simulink library "lib_mtpa_reference_current_generator"  (R2023a)
settings: Solver=VariableStepAuto  StartTime=0.0  StopTime=10.0  RelTol=1e-3
libraries: lib_conversion x14, lib_dynamic_saturator x2, lib_square_root x2, simulink x1
settings Model: Creator=cav2ofo  LastModifiedBy=lenovo
settings OptimizationCC: ReuseModelBlockBuffer=off

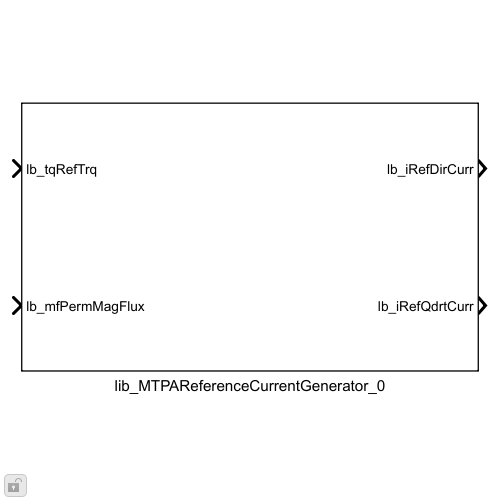
[thumbnail: Simulink's stored preview of the top-level diagram]
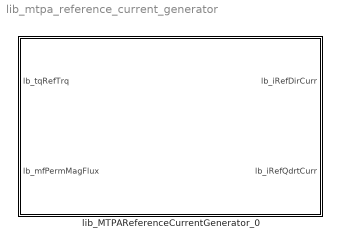
== system lib_mtpa_reference_current_generator ==
  lib_MTPAReferenceCurrentGenerator_0 : Subsystem  mask{lb_parPolePairNum=5, lb_parPermMagFlux=2e-3, lb_parMagTempCoef=-1e-3, lb_parDirIndc=1e-5, lb_parQdrtIndc=1e-5, lb_parMaxPhsCurr=50, lb_parDmgzFact=1, lb_parMaxOperTrq=1, lb_parMinOperTrq=-1, lb_parTrqSampNum=60, lb_parMaxOperTemp=140, lb_parMinOperTemp=-20, lb_parTempSampNum=20, lb_parOutpDataType=Inherit: Inherit via back propagation}
      mask prompts: lb_parPolePairNum "Pole pairs number [-]:"; lb_parPermMagFlux "Permanent magnet flux at 20[oC]:"; lb_parMagTempCoef "Magnet temperature coefficient [1/K]:"; lb_parDirIndc "Direct inductance [H]:"; lb_parQdrtIndc "Quadrature inductance [H]:"; lb_parMaxPhsCurr "Maximum phase current [A]:"; lb_parDmgzFact "Demagnetization factor [-]:"; lb_parMaxOperTrq "Maximum operating torque [Nm]:"; lb_parMinOperTrq "Minimum operating torque [Nm]:"; lb_parTrqSampNum "Torque samplings number:"; lb_parMaxOperTemp "Maximum operating temperature [oC]:"; lb_parMinOperTemp "Minimum operating temperature [oC]:"; lb_parTempSampNum "Temperature samplings number:"; lb_parOutpDataType "Output data type:"
      mask init:
      | temp.PermMagFlux_scl = double(lb_parPermMagFlux);  % [Vs] Permanent magnet flux at 20°C
      | temp.Ld_scl = double(lb_parDirIndc);  % [H] Direct inductance
      | temp.Lq_scl = double(lb_parQdrtIndc);  % [H] Quadrature inductance
      | temp.Npp_scl = double(lb_parPolePairNum);  % Number of pole pairs
      | temp.TmpCoeff_scl = double(lb_parMagTempCoef);  % [1/K] Temperature coefficient of permanent magnet
      | temp.IPhaseMax_scl = double(lb_parMaxPhsCurr);  % [A] Max phase current
      | 
      | % Define torque data
      | temp.Trq_arr = linspace(lb_parMinOperTrq,lb_parMaxOperTrq,lb_parTrqSampNum);  % [Nm] Reference values of electric torque
      | temp.NewTrqStep_scl = 2^(ceil(log2((lb_parMaxOperTrq-lb_parMinOperTrq)/(lb_parTrqSampNum-1))));
      | temp.NewMaxTrq_scl = lb_parMinOperTrq + temp.NewTrqStep_scl*(lb_parTrqSampNum-1);
      | temp.Trq_arr = (lb_parMinOperTrq:temp.NewTrqStep_scl:temp.NewMaxTrq_scl);
      | 
      | % Define temperature/permanent magnet flux data
      | temp.MaxPermMagFlux_scl = temp.PermMagFlux_scl*(1+temp.TmpCoeff_scl*(lb_parMinOperTemp-20));
      | temp.MinPermMagFlux_scl = temp.PermMagFlux_scl*(1+temp.TmpCoeff_scl*(lb_parMaxOperTemp-20));
      | temp.PermMagFlux_arr = linspace(temp.MinPermMagFlux_scl,temp.MaxPermMagFlux_scl,lb_parTempSampNum);
      | temp.NewPermMagFluxStep_scl = 2^(ceil(log2((temp.MaxPermMagFlux_scl-temp.MinPermMagFlux_scl)/(lb_parTempSampNum-1))));
      | temp.NewMaxPermMagFlux_scl = temp.MinPermMagFlux_scl + temp.NewPermMagFluxStep_scl*(lb_parTempSampNum-1);
      | temp.PermMagFlux_arr = linspace(temp.MinPermMagFlux_scl,temp.NewMaxPermMagFlux_scl,lb_parTempSampNum);
      | 
      | temp.IdMTPA_mat = zeros(lb_parTrqSampNum,lb_parTempSampNum);  % [A] Initialization of MTPA LUT
      | 
      | 
      | 
      | for ii = 1:lb_parTrqSampNum
      | 
      |     for jj = 1:lb_parTempSampNum
      | 
      |         % The following quartic equation represents the Maximum Torque Per Ampere
      |         % control strategy. The solution returns the direct current adsdsadsdds
      |         % corresponding to a given electric torque.
      | 
      |         temp.idMTPA_fun = @(id) 1e10*(9*temp.Npp_scl^2*(temp.Lq_scl-temp.Ld_scl)^3*id.^4 + ...
      |             - 27*temp.Npp_scl^2*temp.PermMagFlux_arr(jj)*(temp.Lq_scl-temp.Ld_scl)^2*id.^3 + ...
      |             27*temp.Npp_scl^2*temp.PermMagFlux_arr(jj)^2*(temp.Lq_scl-temp.Ld_scl)*id.^2 + ...
      |             - 9*temp.Npp_scl^2*temp.PermMagFlux_arr(jj)^3*id + ...
      |             - 4*(temp.Lq_scl-temp.Ld_scl)*temp.Trq_arr(ii)^2);
      | 
      |         if jj == 1 || jj == 2
      |             temp.IdMTPA_mat(ii,jj) = real(fzero(temp.idMTPA_fun,-1e-1));
      |         else
      |             temp.IdMTPA_mat(ii,jj) = fzero(temp.idMTPA_fun,temp.IdMTPA_mat(ii,jj-1));
      |         end
      | 
      |     end
      | end
      | 
      | lb_parMTPATrqDataFrstVal = temp.Trq_arr(1);
      | lb_parMTPATrqDataStepVal = temp.NewTrqStep_scl;
      | lb_parMTPAPermMagFluxDataFrstVal = temp.PermMagFlux_arr(1);
      | lb_parMTPAPermMagFluxDataStepVal = temp.NewPermMagFluxStep_scl;
      | lb_parMTPA2DLktMtrx = temp.IdMTPA_mat;
      | 
      | 
      | 
      | clear temp
      settings: LibrarySourceBlock=lib_reference_current_generator/lib_ReferenceCurrentGenerator_0
      mask DialogControl DescGroupVar Prompt: VHIT control library
      mask DialogControl DescTextVar Prompt: Reference current generator
      mask DialogControl Container4 Prompt: Lookup table parameters
      mask DialogControl Container3 Prompt: Data type

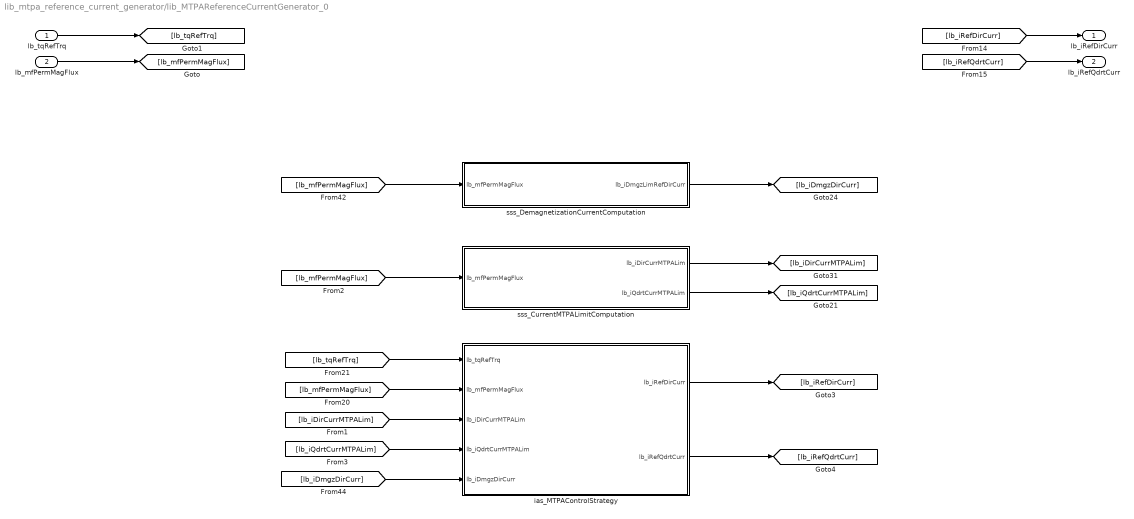
== system lib_mtpa_reference_current_generator/lib_MTPAReferenceCurrentGenerator_0 ==
  lb_tqRefTrq : Inport
  lb_mfPermMagFlux : Inport  Port=2
  ias_MTPAControlStrategy : Subsystem  TreatAsAtomicUnit=on
  sss_CurrentMTPALimitComputation : Subsystem
  sss_DemagnetizationCurrentComputation : Subsystem
  lb_iRefDirCurr : Outport
  lb_iRefQdrtCurr : Outport  Port=2
  wires:
  [lb_mfPermMagFlux] -> sss_DemagnetizationCurrentComputation/1(lb_mfPermMagFlux)
  lb_mfPermMagFlux/1 -> [lb_mfPermMagFlux]
  ias_MTPAControlStrategy/1(lb_iRefDirCurr) -> [lb_iRefDirCurr]
  lb_tqRefTrq/1 -> [lb_tqRefTrq]
  [lb_iRefDirCurr] -> lb_iRefDirCurr/1
  [lb_mfPermMagFlux] -> ias_MTPAControlStrategy/2(lb_mfPermMagFlux)
  [lb_iDirCurrMTPALim] -> ias_MTPAControlStrategy/3(lb_iDirCurrMTPALim)
  ias_MTPAControlStrategy/2(lb_iRefQdrtCurr) -> [lb_iRefQdrtCurr]
  sss_CurrentMTPALimitComputation/2(lb_iQdrtCurrMTPALim) -> [lb_iQdrtCurrMTPALim]
  [lb_iRefQdrtCurr] -> lb_iRefQdrtCurr/1
  [lb_tqRefTrq] -> ias_MTPAControlStrategy/1(lb_tqRefTrq)
  sss_CurrentMTPALimitComputation/1(lb_iDirCurrMTPALim) -> [lb_iDirCurrMTPALim]
  [lb_iQdrtCurrMTPALim] -> ias_MTPAControlStrategy/4(lb_iQdrtCurrMTPALim)
  [lb_mfPermMagFlux] -> sss_CurrentMTPALimitComputation/1(lb_mfPermMagFlux)
  [lb_iDmgzDirCurr] -> ias_MTPAControlStrategy/5(lb_iDmgzDirCurr)
  sss_DemagnetizationCurrentComputation/1(lb_iDmgzLimRefDirCurr) -> [lb_iDmgzDirCurr]

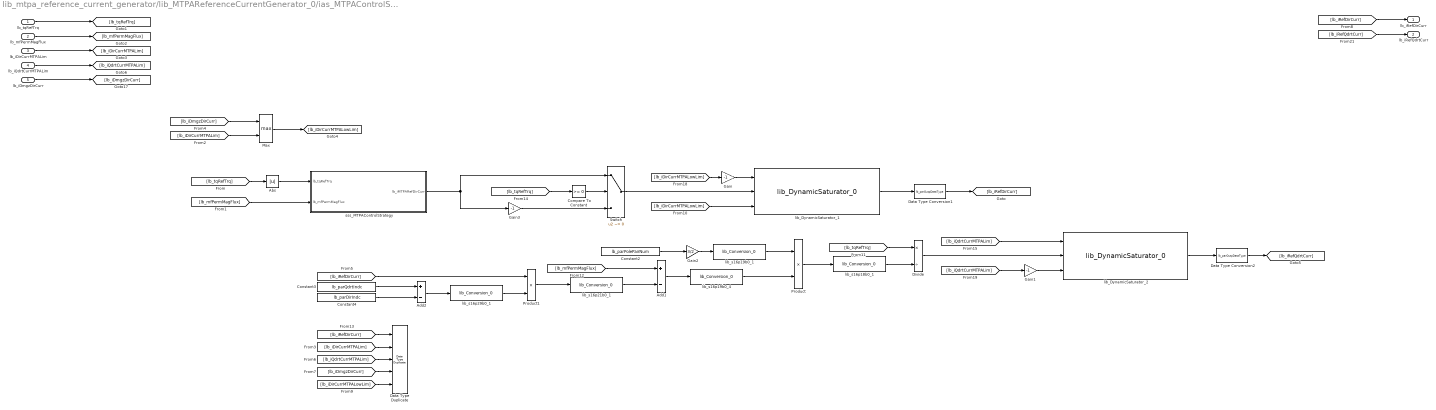
== system lib_mtpa_reference_current_generator/lib_MTPAReferenceCurrentGenerator_0/ias_MTPAControlStrategy ==
  lb_tqRefTrq : Inport
  lb_mfPermMagFlux : Inport  Port=2
  lb_iDirCurrMTPALim : Inport  Port=3
  lb_iQdrtCurrMTPALim : Inport  Port=4
  lb_iDmgzDirCurr : Inport  Port=5
  Abs : Abs  SaturateOnIntegerOverflow=off
  Add1 : Sum  Inputs=+-  OutDataTypeStr=Inherit: Inherit via back propagation  RndMeth=Simplest
  Add2 : Sum  Inputs=+-  OutDataTypeStr=Inherit: Inherit via back propagation  RndMeth=Simplest
  Compare To Constant : simulink/Logic and Bit Operations/Compare To Constant  relop=>=  const=0  OutDataTypeStr=boolean
  Constant2 : Constant  Value=lb_parPolePairNum
  Constant3 : Constant  Value=lb_parQdrtIndc
  Constant4 : Constant  Value=lb_parDirIndc
  Data Type Duplicate : DataTypeDuplicate  NumInputPorts=5
  Data Type Conversion1 : DataTypeConversion  OutDataTypeStr=lb_parOutpDataType  SaturateOnIntegerOverflow=off  RndMeth=Floor
  Data Type Conversion2 : DataTypeConversion  OutDataTypeStr=lb_parOutpDataType  SaturateOnIntegerOverflow=off  RndMeth=Floor
  Divide : Product  Inputs=*/  OutDataTypeStr=Inherit: Inherit via back propagation  RndMeth=Simplest
  Gain : Gain  Gain=-1  OutDataTypeStr=Inherit: Inherit via back propagation  RndMeth=Simplest
  Gain1 : Gain  Gain=-1  OutDataTypeStr=Inherit: Inherit via back propagation  RndMeth=Simplest
  Gain2 : Gain  Gain=3/2  OutDataTypeStr=Inherit: Inherit via back propagation  RndMeth=Simplest
  Gain3 : Gain  Gain=-1  OutDataTypeStr=Inherit: Same as input
  Max : MinMax  Function=max  Inputs=2  OutDataTypeStr=Inherit: Inherit via back propagation
  Product : Product  OutDataTypeStr=Inherit: Inherit via back propagation  RndMeth=Simplest
  Product1 : Product  OutDataTypeStr=Inherit: Inherit via back propagation  RndMeth=Simplest
  Switch : Switch  Criteria=u2 ~= 0  SaturateOnIntegerOverflow=off  InputSameDT=off
  lib_DynamicSaturator_1 : lib_dynamic_saturator/lib_DynamicSaturator_0
  lib_DynamicSaturator_2 : lib_dynamic_saturator/lib_DynamicSaturator_0
  lib_s16p18b0_1 : lib_conversion/lib_Conversion_0  lb_parDataType=fixdt(1,16,2^-18,0)  lb_parOutpMaxVal=[]  lb_parOutpMinVal=[]  lb_parSatFlag=off
  lib_s16p19b0_1 : lib_conversion/lib_Conversion_0  lb_parDataType=fixdt(0,16,10^-3,0)  lb_parOutpMaxVal=[]  lb_parOutpMinVal=[]  lb_parSatFlag=off
  lib_s16p19b0_4 : lib_conversion/lib_Conversion_0  lb_parDataType=fixdt(1,16,2^-19,0)  lb_parOutpMaxVal=[]  lb_parOutpMinVal=[]  lb_parSatFlag=off
  lib_s16p21b0_1 : lib_conversion/lib_Conversion_0  lb_parDataType=fixdt(1,16,2^-21,0)  lb_parOutpMaxVal=[]  lb_parOutpMinVal=[]  lb_parSatFlag=off
  lib_s16p29b0_1 : lib_conversion/lib_Conversion_0  lb_parDataType=fixdt(1,16,2^-29,0)  lb_parOutpMaxVal=[]  lb_parOutpMinVal=[]  lb_parSatFlag=off
  sss_MTPAControlStrategy : Subsystem
  lb_iRefDirCurr : Outport
  lb_iRefQdrtCurr : Outport  Port=2
  wires:
  [lb_iRefDirCurr] -> Data Type Duplicate/1
  [lb_iDirCurrMTPALowLim] -> Data Type Duplicate/5
  [lb_iQdrtCurrMTPALim] -> Data Type Duplicate/3
  [lb_iDmgzDirCurr] -> Data Type Duplicate/4
  [lb_iDirCurrMTPALim] -> Data Type Duplicate/2
  [lb_iRefDirCurr] -> lb_iRefDirCurr/1
  [lb_iRefQdrtCurr] -> lb_iRefQdrtCurr/1
  lib_s16p19b0_1/1 -> Product/1
  Gain2/1 -> lib_s16p19b0_1/1
  lb_tqRefTrq/1 -> [lb_tqRefTrq]
  lb_mfPermMagFlux/1 -> [lb_mfPermMagFlux]
  [lb_tqRefTrq] -> Abs/1
  [lb_mfPermMagFlux] -> sss_MTPAControlStrategy/2(lb_mfPermMagFlux)
  [lb_iDirCurrMTPALowLim] -> Gain/1
  lib_DynamicSaturator_1/1 -> Data Type Conversion1/1
  Data Type Conversion1/1 -> [lb_iRefDirCurr]
  Product/1 -> lib_s16p18b0_1/1
  lib_s16p19b0_4/1 -> Product/2
  Add1/1 -> lib_s16p19b0_4/1
  lib_s16p21b0_1/1 -> Add1/2
  lib_s16p18b0_1/1 -> Divide/2
  lib_s16p29b0_1/1 -> Product1/2
  Product1/1 -> lib_s16p21b0_1/1
  [lb_tqRefTrq] -> Divide/1
  [lb_mfPermMagFlux] -> Add1/1
  [lb_iRefDirCurr] -> Product1/1
  Constant3/1 -> Add2/1
  Constant2/1 -> Gain2/1
  Constant4/1 -> Add2/2
  Add2/1 -> lib_s16p29b0_1/1
  [lb_iQdrtCurrMTPALim] -> Gain1/1
  Data Type Conversion2/1 -> [lb_iRefQdrtCurr]
  lib_DynamicSaturator_2/1 -> Data Type Conversion2/1
  [lb_iQdrtCurrMTPALim] -> lib_DynamicSaturator_2/1
  Divide/1 -> lib_DynamicSaturator_2/2
  lb_iDirCurrMTPALim/1 -> [lb_iDirCurrMTPALim]
  lb_iQdrtCurrMTPALim/1 -> [lb_iQdrtCurrMTPALim]
  lb_iDmgzDirCurr/1 -> [lb_iDmgzDirCurr]
  [lb_iDirCurrMTPALim] -> Max/2
  [lb_iDmgzDirCurr] -> Max/1
  Max/1 -> [lb_iDirCurrMTPALowLim]
  [lb_iDirCurrMTPALowLim] -> lib_DynamicSaturator_1/3
  Gain/1 -> lib_DynamicSaturator_1/1
  Gain1/1 -> lib_DynamicSaturator_2/3
  Abs/1 -> sss_MTPAControlStrategy/1(lb_tqRefTrq)
  [lb_tqRefTrq] -> Compare To Constant/1
  Compare To Constant/1 -> Switch/2
  Gain3/1 -> Switch/3
  Switch/1 -> lib_DynamicSaturator_1/2
  sss_MTPAControlStrategy/1(lb_iMTPARefDirCurr) -> Gain3/1, Switch/1

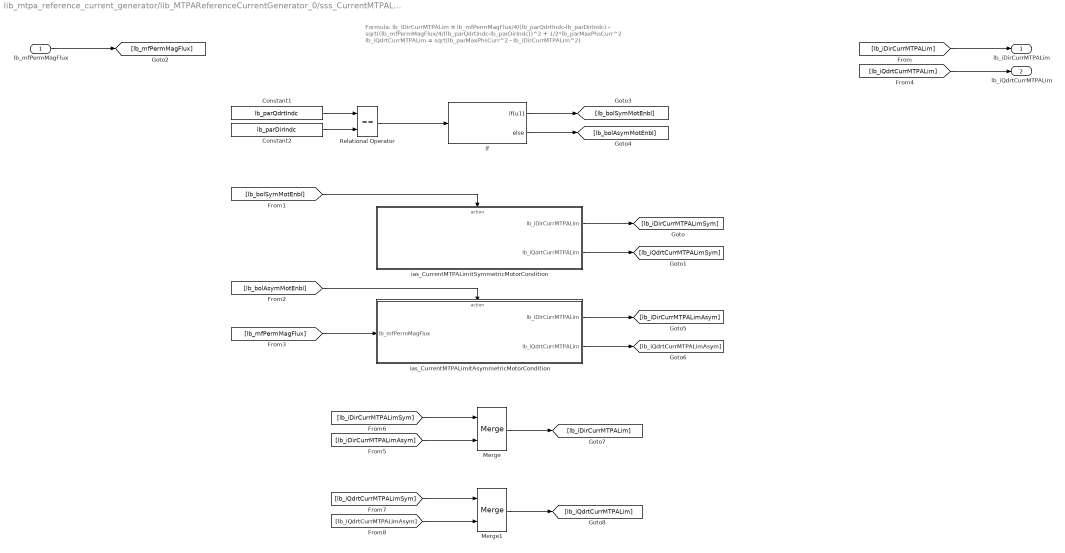
== system lib_mtpa_reference_current_generator/lib_MTPAReferenceCurrentGenerator_0/sss_CurrentMTPALimitComputation ==
  note: Formula:
      | lb_iDirCurrMTPALim = lb_mfPermMagFlux/4/(lb_parQdrtIndc-lb_parDirIndc) - sqrt((lb_mfPermMagFlux/4/(lb_parQdrtIndc-lb_parDirIndc))^2 + 1/2*lb_parMaxPhsCurr^2
      | lb_iQdrtCurrMTPALim = sqrt(lb_parMaxPhsCurr^2 - lb_iDirCurrMTPALim^2)
  lb_mfPermMagFlux : Inport
  Constant1 : Constant  Value=lb_parQdrtIndc
  Constant2 : Constant  Value=lb_parDirIndc
  If : If  IfExpression=u1
  Merge : Merge
  Merge1 : Merge
  Relational Operator : RelationalOperator  Operator===  OutDataTypeStr=boolean  RndMeth=Simplest  InputSameDT=off
  ias_CurrentMTPALimitAsymmetricMotorCondition : Subsystem  TreatAsAtomicUnit=on
  ias_CurrentMTPALimitSymmetricMotorCondition : Subsystem  TreatAsAtomicUnit=on
  lb_iDirCurrMTPALim : Outport
  lb_iQdrtCurrMTPALim : Outport  Port=2
  wires:
  Merge1/1 -> [lb_iQdrtCurrMTPALim]
  Merge/1 -> [lb_iDirCurrMTPALim]
  [lb_iQdrtCurrMTPALimAsym] -> Merge1/2
  [lb_iQdrtCurrMTPALimSym] -> Merge1/1
  [lb_iDirCurrMTPALimSym] -> Merge/1
  [lb_iDirCurrMTPALimAsym] -> Merge/2
  [lb_mfPermMagFlux] -> ias_CurrentMTPALimitAsymmetricMotorCondition/1(lb_mfPermMagFlux)
  ias_CurrentMTPALimitAsymmetricMotorCondition/2(lb_iQdrtCurrMTPALim) -> [lb_iQdrtCurrMTPALimAsym]
  ias_CurrentMTPALimitAsymmetricMotorCondition/1(lb_iDirCurrMTPALim) -> [lb_iDirCurrMTPALimAsym]
  ias_CurrentMTPALimitSymmetricMotorCondition/2(lb_iQdrtCurrMTPALim) -> [lb_iQdrtCurrMTPALimSym]
  ias_CurrentMTPALimitSymmetricMotorCondition/1(lb_iDirCurrMTPALim) -> [lb_iDirCurrMTPALimSym]
  [lb_bolAsymMotEnbl] -> ias_CurrentMTPALimitAsymmetricMotorCondition/Action
  [lb_bolSymMotEnbl] -> ias_CurrentMTPALimitSymmetricMotorCondition/Action
  If/2 -> [lb_bolAsymMotEnbl]
  If/1 -> [lb_bolSymMotEnbl]
  Relational Operator/1 -> If/1
  Constant2/1 -> Relational Operator/2
  Constant1/1 -> Relational Operator/1
  [lb_iDirCurrMTPALim] -> lb_iDirCurrMTPALim/1
  [lb_iQdrtCurrMTPALim] -> lb_iQdrtCurrMTPALim/1
  lb_mfPermMagFlux/1 -> [lb_mfPermMagFlux]

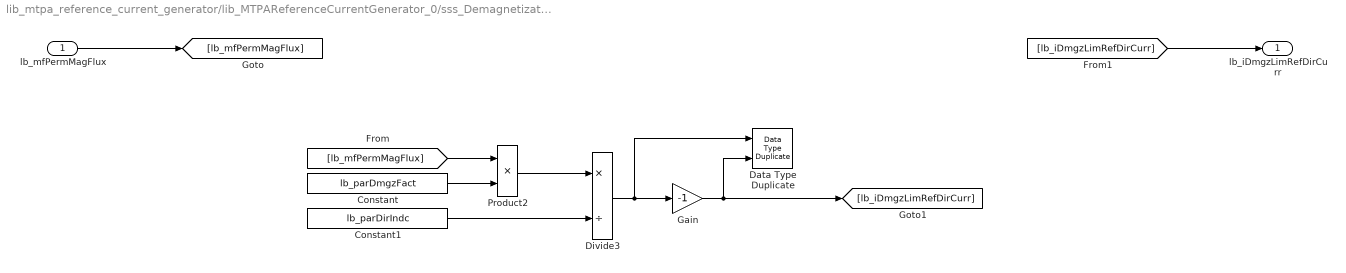
== system lib_mtpa_reference_current_generator/lib_MTPAReferenceCurrentGenerator_0/sss_DemagnetizationCurrentComputation ==
  lb_mfPermMagFlux : Inport
  Constant : Constant  Value=lb_parDmgzFact
  Constant1 : Constant  Value=lb_parDirIndc
  Data Type Duplicate : DataTypeDuplicate
  Divide3 : Product  Inputs=*/  OutDataTypeStr=Inherit: Inherit via back propagation  RndMeth=Simplest
  Gain : Gain  Gain=-1  OutDataTypeStr=Inherit: Inherit via back propagation  RndMeth=Simplest
  Product2 : Product  RndMeth=Simplest  OutDataTypeStr=Inherit: Same as first input
  lb_iDmgzLimRefDirCurr : Outport
  wires:
  Divide3/1 -> Gain/1, Data Type Duplicate/1
  Product2/1 -> Divide3/1
  [lb_mfPermMagFlux] -> Product2/1
  Gain/1 -> [lb_iDmgzLimRefDirCurr], Data Type Duplicate/2
  Constant/1 -> Product2/2
  lb_mfPermMagFlux/1 -> [lb_mfPermMagFlux]
  [lb_iDmgzLimRefDirCurr] -> lb_iDmgzLimRefDirCurr/1
  Constant1/1 -> Divide3/2

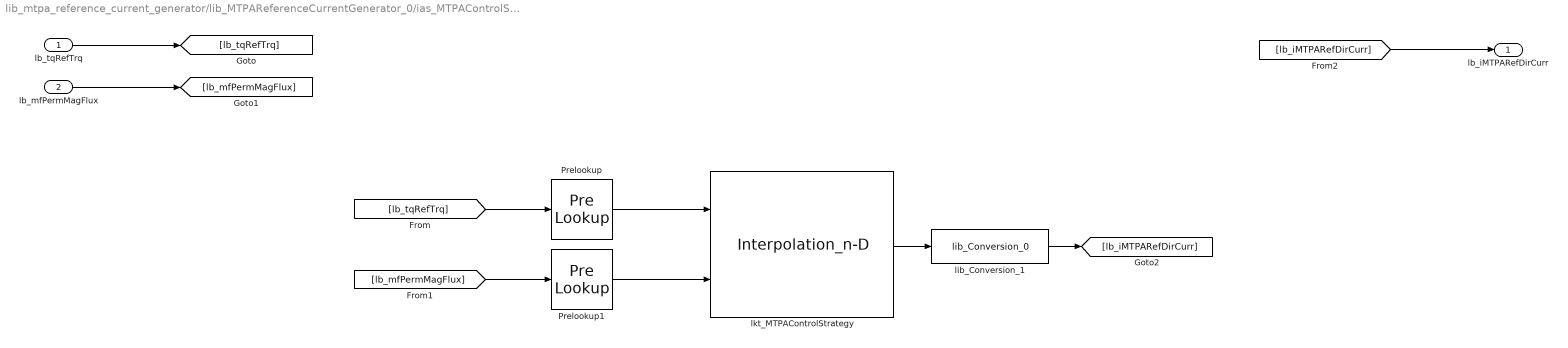
== system lib_mtpa_reference_current_generator/lib_MTPAReferenceCurrentGenerator_0/ias_MTPAControlStrategy/sss_MTPAControlStrategy ==
  lb_tqRefTrq : Inport
  lb_mfPermMagFlux : Inport  Port=2
  Prelookup : PreLookup  BreakpointsData=[10:10:110]  BreakpointsSpecification=Even spacing  BreakpointsNumPoints=lb_parTrqSampNum  BreakpointsFirstPoint=lb_parMTPATrqDataFrstVal  BreakpointsSpacing=lb_parMTPATrqDataStepVal  OutputSelection=Index and fraction as bus  RemoveProtectionInput=on  IndexDataTypeStr=uint16  FractionDataTypeStr=fixdt(0,16,2^-15,0)  RndMeth=Simplest
  Prelookup1 : PreLookup  BreakpointsData=[10:10:110]  BreakpointsSpecification=Even spacing  BreakpointsNumPoints=lb_parTempSampNum  BreakpointsFirstPoint=lb_parMTPAPermMagFluxDataFrstVal  BreakpointsSpacing=lb_parMTPAPermMagFluxDataStepVal  OutputSelection=Index and fraction as bus  RemoveProtectionInput=on  IndexDataTypeStr=uint16  FractionDataTypeStr=fixdt(0,16,2^-15,0)  RndMeth=Simplest
  lib_Conversion_1 : lib_conversion/lib_Conversion_0  lb_parDataType=lb_parOutpDataType  lb_parOutpMaxVal=[]  lb_parOutpMinVal=[]  lb_parSatFlag=off
  lkt_MTPAControlStrategy : Interpolation_n-D  Table=lb_parMTPA2DLktMtrx  ExtrapMethod=Clip  RequireIndexFractionAsBus=on  RemoveProtectionIndex=on  OutDataTypeStr=Inherit: Inherit via back propagation  InternalRulePriority=Speed  RndMeth=Simplest
      settings: InputPortMap=u0,u1
  lb_iMTPARefDirCurr : Outport
  wires:
  lb_tqRefTrq/1 -> [lb_tqRefTrq]
  lb_mfPermMagFlux/1 -> [lb_mfPermMagFlux]
  [lb_tqRefTrq] -> Prelookup/1
  [lb_mfPermMagFlux] -> Prelookup1/1
  Prelookup/1 -> lkt_MTPAControlStrategy/1
  Prelookup1/1 -> lkt_MTPAControlStrategy/2
  lkt_MTPAControlStrategy/1 -> lib_Conversion_1/1
  [lb_iMTPARefDirCurr] -> lb_iMTPARefDirCurr/1
  lib_Conversion_1/1 -> [lb_iMTPARefDirCurr]

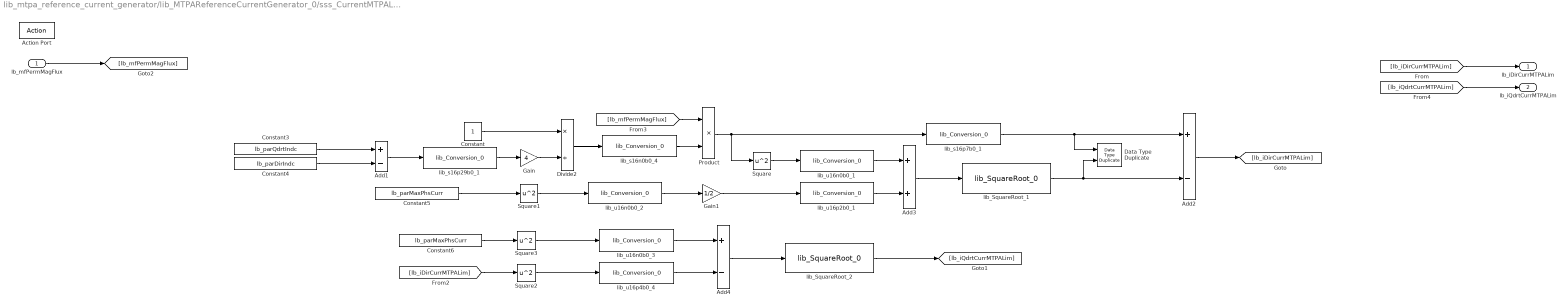
== system lib_mtpa_reference_current_generator/lib_MTPAReferenceCurrentGenerator_0/sss_CurrentMTPALimitComputation/ias_CurrentMTPALimitAsymmetricMotorCondition ==
  lb_mfPermMagFlux : Inport
  Action Port : ActionPort
  Add1 : Sum  Inputs=+-  OutDataTypeStr=Inherit: Inherit via back propagation  RndMeth=Simplest
  Add2 : Sum  Inputs=+-  OutDataTypeStr=Inherit: Inherit via back propagation  RndMeth=Simplest
  Add3 : Sum  RndMeth=Simplest  OutDataTypeStr=Inherit: Same as first input
  Add4 : Sum  Inputs=+-  RndMeth=Simplest  OutDataTypeStr=Inherit: Same as first input
  Constant : Constant  OutDataTypeStr=uint16
  Constant3 : Constant  Value=lb_parQdrtIndc
  Constant4 : Constant  Value=lb_parDirIndc
  Constant5 : Constant  Value=lb_parMaxPhsCurr
  Constant6 : Constant  Value=lb_parMaxPhsCurr
  Data Type Duplicate : DataTypeDuplicate
  Divide2 : Product  Inputs=*/  OutDataTypeStr=Inherit: Inherit via back propagation  RndMeth=Simplest
  Gain : Gain  Gain=4  RndMeth=Simplest  OutDataTypeStr=Inherit: Same as input
  Gain1 : Gain  Gain=1/2  OutDataTypeStr=Inherit: Inherit via back propagation  RndMeth=Simplest
  Product : Product  OutDataTypeStr=Inherit: Inherit via back propagation
  Square{,1..3} (4 alike) : Math  Operator=square  SignedPower=on  OutDataTypeStr=Inherit: Inherit via back propagation  RndMeth=Simplest
  lib_SquareRoot_1 : lib_square_root/lib_SquareRoot_0  lb_parLktSize=1024  lb_parInpDataType=uint16  lb_parOutpDataType=Inherit: Inherit via back propagation
  lib_SquareRoot_2 : lib_square_root/lib_SquareRoot_0  lb_parLktSize=128  lb_parInpDataType=uint16  lb_parOutpDataType=Inherit: Inherit via back propagation
  lib_s16n0b0_4 : lib_conversion/lib_Conversion_0  lb_parDataType=uint32  lb_parOutpMaxVal=[]  lb_parOutpMinVal=[]  lb_parSatFlag=off
  lib_s16p29b0_1 : lib_conversion/lib_Conversion_0  lb_parDataType=fixdt(1,16,2^-29,0)  lb_parOutpMaxVal=[]  lb_parOutpMinVal=[]  lb_parSatFlag=off
  lib_s16p7b0_1 : lib_conversion/lib_Conversion_0  lb_parDataType=fixdt(1,16,2^-7,0)  lb_parOutpMaxVal=[]  lb_parOutpMinVal=[]  lb_parSatFlag=off
  lib_u16n0b0_1 : lib_conversion/lib_Conversion_0  lb_parDataType=uint16  lb_parOutpMaxVal=[]  lb_parOutpMinVal=[]  lb_parSatFlag=off
  lib_u16n0b0_2 : lib_conversion/lib_Conversion_0  lb_parDataType=uint16  lb_parOutpMaxVal=[]  lb_parOutpMinVal=[]  lb_parSatFlag=off
  lib_u16n0b0_3 : lib_conversion/lib_Conversion_0  lb_parDataType=uint16  lb_parOutpMaxVal=[]  lb_parOutpMinVal=[]  lb_parSatFlag=off
  lib_u16p2b0_1 : lib_conversion/lib_Conversion_0  lb_parDataType=fixdt(0,16,2^-2,0)  lb_parOutpMaxVal=[]  lb_parOutpMinVal=[]  lb_parSatFlag=off
  lib_u16p4b0_4 : lib_conversion/lib_Conversion_0  lb_parDataType=fixdt(0,16,2^-4,0)  lb_parOutpMaxVal=[]  lb_parOutpMinVal=[]  lb_parSatFlag=off
  lb_iDirCurrMTPALim : Outport
  lb_iQdrtCurrMTPALim : Outport  Port=2
  wires:
  [lb_iDirCurrMTPALim] -> lb_iDirCurrMTPALim/1
  [lb_iQdrtCurrMTPALim] -> lb_iQdrtCurrMTPALim/1
  lb_mfPermMagFlux/1 -> [lb_mfPermMagFlux]
  Square3/1 -> lib_u16n0b0_3/1
  Square2/1 -> lib_u16p4b0_4/1
  lib_u16p4b0_4/1 -> Add4/2
  lib_s16p29b0_1/1 -> Gain/1
  lib_SquareRoot_2/1 -> [lb_iQdrtCurrMTPALim]
  lib_s16p7b0_1/1 -> Data Type Duplicate/1, Add2/1
  Add4/1 -> lib_SquareRoot_2/1
  Product/1 -> lib_s16p7b0_1/1, Square/1
  lib_u16p2b0_1/1 -> Add3/2
  Add3/1 -> lib_SquareRoot_1/1
  Constant6/1 -> Square3/1
  Constant5/1 -> Square1/1
  Constant4/1 -> Add1/2
  lib_u16n0b0_3/1 -> Add4/1
  lib_u16n0b0_1/1 -> Add3/1
  Gain1/1 -> lib_u16p2b0_1/1
  Add1/1 -> lib_s16p29b0_1/1
  [lb_iDirCurrMTPALim] -> Square2/1
  Square/1 -> lib_u16n0b0_1/1
  Add2/1 -> [lb_iDirCurrMTPALim]
  Constant3/1 -> Add1/1
  lib_SquareRoot_1/1 -> Data Type Duplicate/2, Add2/2
  lib_u16n0b0_2/1 -> Gain1/1
  Square1/1 -> lib_u16n0b0_2/1
  Gain/1 -> Divide2/2
  Constant/1 -> Divide2/1
  [lb_mfPermMagFlux] -> Product/1
  Divide2/1 -> lib_s16n0b0_4/1
  lib_s16n0b0_4/1 -> Product/2

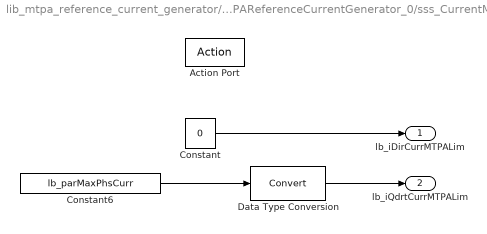
== system lib_mtpa_reference_current_generator/lib_MTPAReferenceCurrentGenerator_0/sss_CurrentMTPALimitComputation/ias_CurrentMTPALimitSymmetricMotorCondition ==
  Action Port : ActionPort
  Constant : Constant  Value=0  OutDataTypeStr=Inherit: Inherit via back propagation
  Constant6 : Constant  Value=lb_parMaxPhsCurr
  Data Type Conversion : DataTypeConversion  SaturateOnIntegerOverflow=off  RndMeth=Floor
  lb_iDirCurrMTPALim : Outport
  lb_iQdrtCurrMTPALim : Outport  Port=2
  wires:
  Data Type Conversion/1 -> lb_iQdrtCurrMTPALim/1
  Constant6/1 -> Data Type Conversion/1
  Constant/1 -> lb_iDirCurrMTPALim/1
